simulink model "Queue_server_Model"  (R2023a)
settings: Solver=VariableStepAuto  StartTime=0.0  StopTime=10.0  RelTol=1e-3
libraries: NSA_DEVS_SINKS_ATOMIC x5, NSA_DEVS_SOURCES_ATOMIC x1, NSA_DEVS_LOGISTICS_ATOMIC x1, NSA_DEVS_LOGISTICS_COUPLED x1
settings Model: Creator=david  LastModifiedBy=david

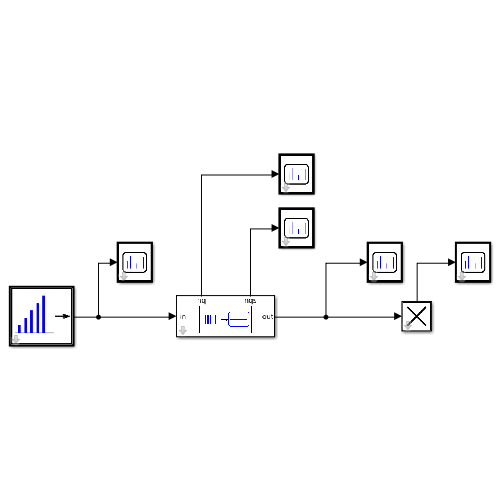
[thumbnail: Simulink's stored preview of the top-level diagram]
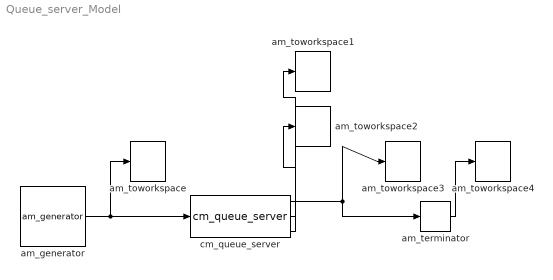
== system Queue_server_Model ==
  am_generator : NSA_DEVS_SOURCES_ATOMIC/am_generator  tG=1  n0=1  nG=20  tau=[0,1]  debug=0
      settings: SourceProductName=NSA_DEVS
  am_terminator : NSA_DEVS_LOGISTICS_ATOMIC/am_terminator  tau=[0,1]  debug=0
      settings: SourceProductName=NSA_DEVS
  am_toworkspace : NSA_DEVS_SINKS_ATOMIC/am_toworkspace  varname="\"genout\""  t0=0  format="\"vector\""  tau=[0,5]  debug=0
      settings: SourceProductName=NSA_DEVS
  am_toworkspace1 : NSA_DEVS_SINKS_ATOMIC/am_toworkspace  varname="\"nq\""  t0=0  format="\"vector\""  tau=[0,5]  debug=0
      settings: SourceProductName=NSA_DEVS
  am_toworkspace2 : NSA_DEVS_SINKS_ATOMIC/am_toworkspace  varname="\"nqs\""  t0=0  format="\"vector\""  tau=[0,5]  debug=0
      settings: SourceProductName=NSA_DEVS
  am_toworkspace3 : NSA_DEVS_SINKS_ATOMIC/am_toworkspace  varname="\"srvout\""  t0=0  format="\"vector\""  tau=[0,5]  debug=0
      settings: SourceProductName=NSA_DEVS
  am_toworkspace4 : NSA_DEVS_SINKS_ATOMIC/am_toworkspace  varname="\"nout\""  t0=0  format="\"vector\""  tau=[0,5]  debug=0
      settings: SourceProductName=NSA_DEVS
  cm_queue_server : NSA_DEVS_LOGISTICS_COUPLED/cm_queue_server  ts=4.5  tau=[0,1]  debug=0
      settings: SourceProductName=NSA_DEVS
  wires:
  am_generator/1 -> am_toworkspace/1, cm_queue_server/1
  cm_queue_server/1 -> am_toworkspace3/1, am_terminator/1
  cm_queue_server/2 -> am_toworkspace1/1
  cm_queue_server/3 -> am_toworkspace2/1
  am_terminator/1 -> am_toworkspace4/1
